simulink model "test"  (R2020a)
settings: Solver=VariableStepAuto  StartTime=0.0  StopTime=10  RelTol=1e-3
values from neighbouring files (symbols this model uses):
  den1 = [1 b*(i+m*l^2)/q1 -(M+m)*m*g*l/q1 -b*m*g*l/q1]    [parameter.m]
  g = 9.8    [parameter.m]
  num1 = [m*l/q1 0]    [parameter.m]
undefined symbols (not defined in the file or in its folder): d, DiscIntNeverNeededParam, I3, mc, ms, R, Ts
libraries: simulink x2, rllib x1
settings Model: Creator=Preload  LastModifiedBy=User
settings DataIOCC: ReturnWorkspaceOutputs=off
settings DebuggingCC: ArithmeticOperatorsInVariantConditions=warning
settings SFSimCC: SimUseLocalCustomCode=off  CustomCodeUndefinedFunction=UseInterfaceOnly
settings RTWCC: RTWUseLocalCustomCode=off

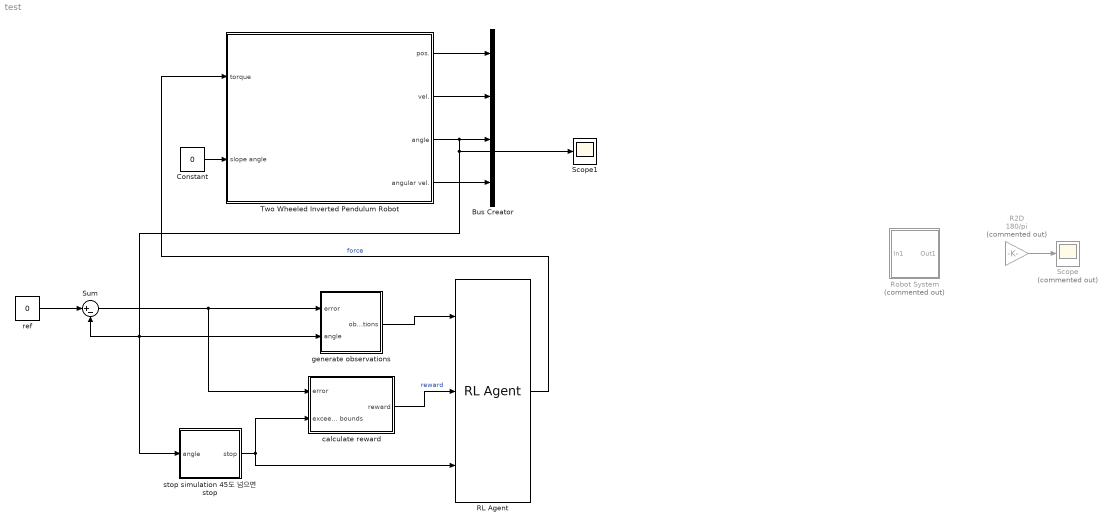
== system test ==
  Bus Creator : BusCreator  Inputs=4
  Constant : Constant  Value=0
  R2D : Gain  Commented=on  Gain=180/pi
  RL Agent : rllib/RL Agent  Agent=agent  ProvideReward=on  ProvideIsDone=on  ProvideCumRwd=off  TreatAsDirectFeedthrough=on  CollectLoggedSignals=on  CollectModelStates=on
  Robot System : Subsystem  Commented=on
  Scope : Scope  Commented=on
  Scope1 : Scope
  Sum : Sum  Inputs=|+-
  Two Wheeled Inverted Pendulum Robot : Subsystem
  calculate reward : Subsystem
  generate observations : Subsystem
  ref : Constant  Value=0
  stop simulation 45도 넘으면 stop : Subsystem
  wires:
  ref/1 -> Sum/1
  R2D/1 -> Scope/1
  RL Agent/1 -> Two Wheeled Inverted Pendulum Robot/1(torque)  "force"
  stop simulation 45도 넘으면 stop/1(stop) -> calculate reward/2(exceeds bounds), RL Agent/3
  calculate reward/1(reward) -> RL Agent/2  "reward"
  Sum/1 -> calculate reward/1(error), generate observations/1(error)
  generate observations/1(observations) -> RL Agent/1
  Constant/1 -> Two Wheeled Inverted Pendulum Robot/2(slope angle)
  Two Wheeled Inverted Pendulum Robot/1(pos.) -> Bus Creator/1
  Two Wheeled Inverted Pendulum Robot/2(vel.) -> Bus Creator/2
  Two Wheeled Inverted Pendulum Robot/3(angle) -> Scope1/1, Sum/2, generate observations/2(angle), stop simulation 45도 넘으면 stop/1(angle), Bus Creator/3
  Two Wheeled Inverted Pendulum Robot/4(angular vel.) -> Bus Creator/4

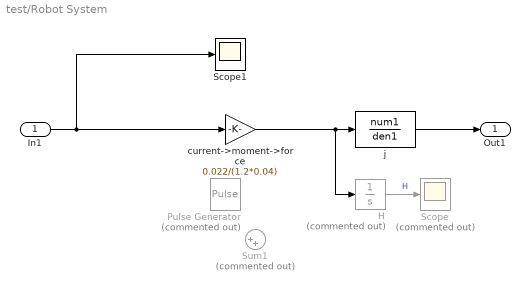
== system test/Robot System ==
  In1 : Inport
  H : Integrator  Commented=on  LimitOutput=on  LowerSaturationLimit=0
  Pulse Generator : DiscretePulseGenerator  Commented=on  PulseType=Time based  Amplitude=10  Period=10  PulseWidth=0.1  PhaseDelay=0.1
  Scope : Scope  Commented=on
  Scope1 : Scope
  Sum1 : Sum  Commented=on  Inputs=|++
  current->moment->force : Gain  Gain=0.022/(1.2*0.04)
  j : TransferFcn  Numerator=num1  Denominator=den1
  Out1 : Outport
  wires:
  In1/1 -> current->moment->force/1, Scope1/1
  j/1 -> Out1/1
  current->moment->force/1 -> H/1, j/1
  H/1 -> Scope/1  "H"

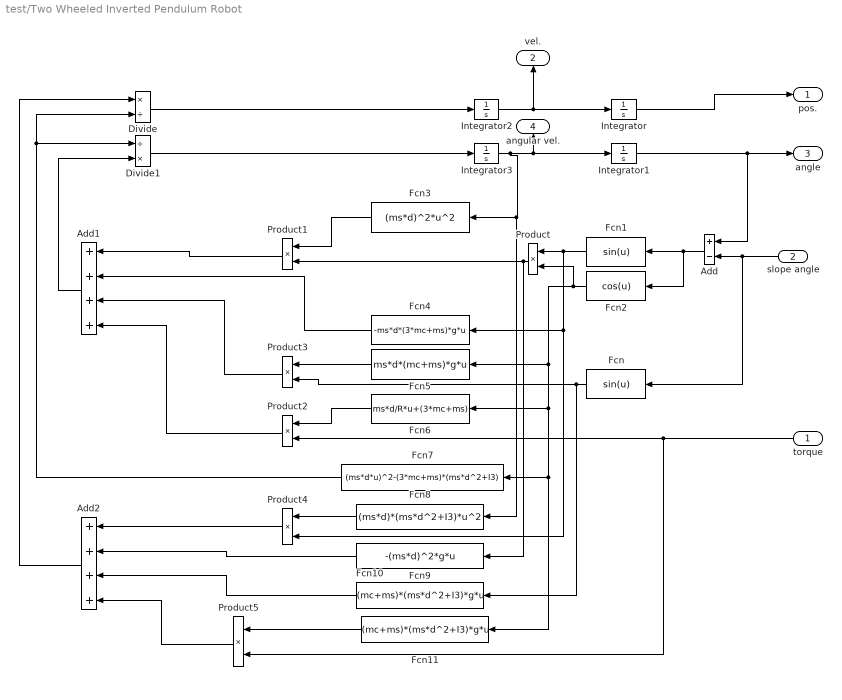
== system test/Two Wheeled Inverted Pendulum Robot ==
  torque : Inport
  slope angle : Inport  Port=2
  Add : Sum  Inputs=+-
  Add1 : Sum  Inputs=++++
  Add2 : Sum  Inputs=++++
  Divide : Product  Inputs=*/
  Divide1 : Product  Inputs=/*
  Fcn : Fcn  Expr=sin(u)
  Fcn1 : Fcn  Expr=sin(u)
  Fcn10 : Fcn  Expr=(mc+ms)*(ms*d^2+I3)*g*u
  Fcn11 : Fcn  Expr=(mc+ms)*(ms*d^2+I3)*g*u
  Fcn2 : Fcn  Expr=cos(u)
  Fcn3 : Fcn  Expr=(ms*d)^2*u^2
  Fcn4 : Fcn  Expr=-ms*d*(3*mc+ms)*g*u
  Fcn5 : Fcn  Expr=ms*d*(mc+ms)*g*u
  Fcn6 : Fcn  Expr=ms*d/R*u+(3*mc+ms)
  Fcn7 : Fcn  Expr=(ms*d*u)^2-(3*mc+ms)*(ms*d^2+I3)
  Fcn8 : Fcn  Expr=(ms*d)*(ms*d^2+I3)*u^2
  Fcn9 : Fcn  Expr=-(ms*d)^2*g*u
  Integrator{,1..3} (4 alike) : Integrator
  Product{,1..5} (6 alike) : Product
  pos. : Outport
  vel. : Outport  Port=2
  angle : Outport  Port=3
  angular vel. : Outport  Port=4
  wires:
  Product4/1 -> Add2/1
  Integrator1/1 -> angle/1, Add/1
  Add/1 -> Fcn2/1, Fcn1/1
  Add1/1 -> Divide1/2
  Integrator3/1 -> Fcn3/1, Fcn8/1, angular vel./1, Integrator1/1
  Divide/1 -> Integrator2/1
  Integrator2/1 -> vel./1, Integrator/1
  Product3/1 -> Add1/3
  Fcn/1 -> Fcn10/1, Product3/2
  Integrator/1 -> pos./1
  Product1/1 -> Add1/1
  Fcn6/1 -> Product2/1
  Fcn1/1 -> Fcn4/1, Product4/2, Product/1
  slope angle/1 -> Fcn/1, Add/2
  torque/1 -> Product2/2, Product5/2
  Fcn7/1 -> Divide/2, Divide1/1
  Fcn2/1 -> Fcn11/1, Fcn7/1, Fcn6/1, Fcn5/1, Product/2
  Product/1 -> Product1/2, Fcn9/1
  Fcn5/1 -> Product3/1
  Divide1/1 -> Integrator3/1
  Product2/1 -> Add1/4
  Fcn3/1 -> Product1/1
  Fcn4/1 -> Add1/2
  Product5/1 -> Add2/4
  Fcn10/1 -> Add2/3
  Fcn8/1 -> Product4/1
  Fcn9/1 -> Add2/2
  Add2/1 -> Divide/1
  Fcn11/1 -> Product5/1

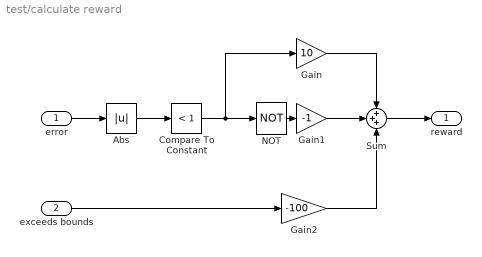
== system test/calculate reward ==
  error : Inport
  exceeds bounds : Inport  Port=2
  Abs : Abs
  Compare To Constant : simulink/Logic and Bit Operations/Compare To Constant  relop=<  const=1  OutDataTypeStr=boolean
  Gain : Gain  Gain=10
  Gain1 : Gain  Gain=-1
  Gain2 : Gain  Gain=-100
  NOT : Logic  Operator=NOT  IconShape=distinctive  AllPortsSameDT=off  OutDataTypeStr=boolean
  Sum : Sum  Inputs=+++  OutDataTypeStr=double
  reward : Outport  VectorParamsAs1DForOutWhenUnconnected=off
  wires:
  Sum/1 -> reward/1
  Compare To Constant/1 -> NOT/1, Gain/1
  NOT/1 -> Gain1/1
  exceeds bounds/1 -> Gain2/1
  Gain/1 -> Sum/1
  error/1 -> Abs/1
  Gain1/1 -> Sum/2
  Gain2/1 -> Sum/3
  Abs/1 -> Compare To Constant/1

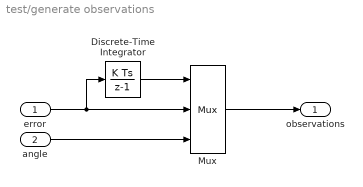
== system test/generate observations ==
  error : Inport
  angle : Inport  Port=2
  Discrete-Time Integrator : DiscreteIntegrator  SampleTime=Ts  ICPrevOutput=DiscIntNeverNeededParam  ICPrevScaledInput=DiscIntNeverNeededParam
  Mux : Mux  Inputs=3
  observations : Outport  VectorParamsAs1DForOutWhenUnconnected=off
  wires:
  angle/1 -> Mux/3
  Discrete-Time Integrator/1 -> Mux/1
  error/1 -> Discrete-Time Integrator/1, Mux/2
  Mux/1 -> observations/1

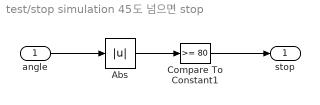
== system test/stop simulation 45도 넘으면 stop ==
  angle : Inport
  Abs : Abs
  Compare To Constant1 : simulink/Logic and Bit Operations/Compare To Constant  relop=>=  const=80  OutDataTypeStr=boolean
  stop : Outport  VectorParamsAs1DForOutWhenUnconnected=off
  wires:
  Compare To Constant1/1 -> stop/1
  Abs/1 -> Compare To Constant1/1
  angle/1 -> Abs/1
